simulink model "ukol_5_model_2"  (R2016a)
settings: Solver=VariableStepAuto  SolverMode=SingleTasking  StartTime=0.0  StopTime=30  MaxStep=1e-2  RelTol=1e-3
undefined symbols (not defined in the file): A, B, C, D, k1, k1_2, k2, k2_2, kI, korekcni_zesileni
settings Model: Creator=tomas  LastModifiedBy=tomas
settings DebuggingCC: SFUnexpectedBacktrackingDiag=error  SFNoUnconditionalDefaultTransitionDiag=error
settings GRTTargetCC: TargetLangStandard=C99 (ISO)  GeneratePreprocessorConditionals=Use local settings
settings ConfigComp: CovMetricSettings=dwe  CovHtmlReporting=off  CovSaveCumulativeToWorkspaceVar=off  CovSaveSingleToWorkspaceVar=off  CovExternalEMLEnable=on

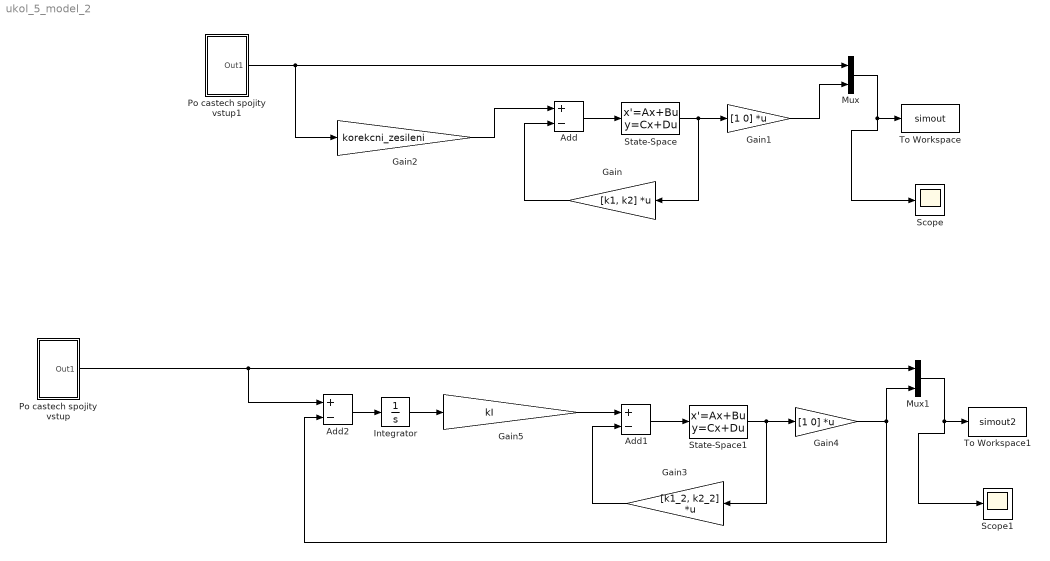
== system ukol_5_model_2 ==
  Add : Sum  Inputs=+-
  Add1 : Sum  Inputs=+-
  Add2 : Sum  Inputs=+-
  Gain : Gain  Gain=[k1, k2]  Multiplication=Matrix(K*u)
  Gain1 : Gain  Gain=[1 0]  Multiplication=Matrix(K*u)
  Gain2 : Gain  Gain=korekcni_zesileni
  Gain3 : Gain  Gain=[k1_2, k2_2]  Multiplication=Matrix(K*u)
  Gain4 : Gain  Gain=[1 0]  Multiplication=Matrix(K*u)
  Gain5 : Gain  Gain=kI
  Integrator : Integrator
  Mux : Mux  Inputs=2
  Mux1 : Mux  Inputs=2
  Po castech spojity vstup : Subsystem
  Po castech spojity vstup1 : Subsystem
  Scope : Scope
  Scope1 : Scope
  State-Space : StateSpace  A=A  B=B  C=C  D=D  X0=0
  State-Space1 : StateSpace  A=A  B=B  C=C  D=D  X0=0
  To Workspace : ToWorkspace  VariableName=simout  SaveFormat=Timeseries  SampleTime=-1
  To Workspace1 : ToWorkspace  VariableName=simout2  SaveFormat=Timeseries  SampleTime=-1
  wires:
  State-Space/1 -> Gain/1, Gain1/1
  Add/1 -> State-Space/1
  Gain/1 -> Add/2
  Gain1/1 -> Mux/2
  Mux/1 -> Scope/1, To Workspace/1
  Gain2/1 -> Add/1
  Gain5/1 -> Add1/1
  Gain4/1 -> Add2/2, Mux1/2
  State-Space1/1 -> Gain3/1, Gain4/1
  Add1/1 -> State-Space1/1
  Mux1/1 -> Scope1/1, To Workspace1/1
  Gain3/1 -> Add1/2
  Integrator/1 -> Gain5/1
  Add2/1 -> Integrator/1
  Po castech spojity vstup/1(Out1) -> Add2/1, Mux1/1
  Po castech spojity vstup1/1(Out1) -> Gain2/1, Mux/1

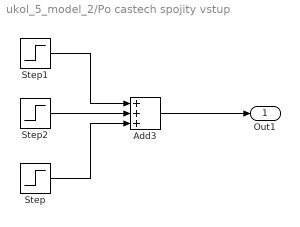
== system ukol_5_model_2/Po castech spojity vstup ==
  Add3 : Sum  Inputs=+++
  Step : Step  SampleTime=0
  Step1 : Step  Time=5  After=-4  SampleTime=0
  Step2 : Step  Time=15  After=8  SampleTime=0
  Out1 : Outport
  wires:
  Step1/1 -> Add3/1
  Add3/1 -> Out1/1
  Step/1 -> Add3/3
  Step2/1 -> Add3/2

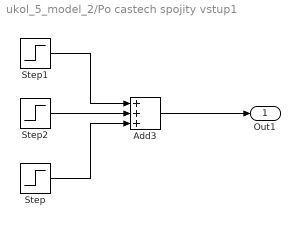
== system ukol_5_model_2/Po castech spojity vstup1 ==
  Add3 : Sum  Inputs=+++
  Step : Step  SampleTime=0
  Step1 : Step  Time=5  After=-4  SampleTime=0
  Step2 : Step  Time=15  After=8  SampleTime=0
  Out1 : Outport
  wires:
  Step2/1 -> Add3/2
  Step/1 -> Add3/3
  Add3/1 -> Out1/1
  Step1/1 -> Add3/1
